simulink model "buck_conv"  (R2020b)
settings: Solver=ode3  StartTime=0.0  StopTime=0.06  FixedStep=1e-7  RelTol=1e-3  EnableMultiTasking=on
undefined symbols (not defined in the file): C, ki, kp, L, R, T, Vin, Vo
libraries: simulink x3
settings Model: Creator=Anandarup  LastModifiedBy=Anandarup
settings DataIOCC: LimitDataPoints=on  SaveFormat=Array  ReturnWorkspaceOutputs=off
settings OptimizationCC: LifeSpan=inf
settings DebuggingCC: SolverPrmCheckMsg=warning  SFUnexpectedBacktrackingDiag=warning  SFNoUnconditionalDefaultTransitionDiag=warning  SFExecutionAtInitializationDiag=none  ArithmeticOperatorsInVariantConditions=warning
settings HardwareCC: ProdBitPerPointer=32  ProdBitPerSizeT=32  ProdBitPerPtrDiffT=32  ProdLargestAtomicFloat=None  ProdIntDivRoundTo=Undefined  ProdEndianess=Unspecified  ProdWordSize=32  ProdHWDeviceType=32-bit Generic
settings ModelReferenceCC: PropagateSignalLabelsOutOfModel=off
settings SFSimCC: SimUseLocalCustomCode=off  CustomCodeUndefinedFunction=UseInterfaceOnly
settings RTWCC: RTWUseLocalCustomCode=off
settings CodeAppCC: StateflowObjectComments=on
settings GRTTargetCC: TargetLangStandard=C89/C90 (ANSI)
settings ConfigComp: CovMetricSettings=dw  CovSaveCumulativeToWorkspaceVar=on  CovSaveSingleToWorkspaceVar=on  CovExternalEMLEnable=off  CovSFcnEnable=off

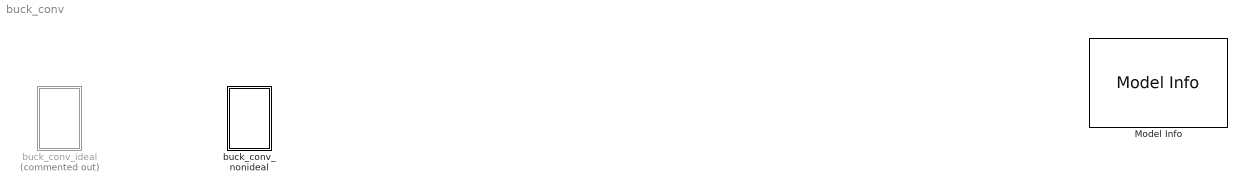
== system buck_conv ==
  Model Info : simulink/Model-Wide Utilities/Model Info  Frame=on  DisplayStringWithTags=|  HorizontalTextAlignment=Center  LeftAlignmentValue=0.5
      | clear;
      | clc;
      | R=5;
      | Vin=24;
      | L=750e-6;
      | C=1.5e-6;
      | Vo=15;
      | kp=20;
      | ki=10;
      | T=1/50e3;
  buck_conv_ideal : Subsystem  Commented=on
  buck_conv_nonideal : Subsystem

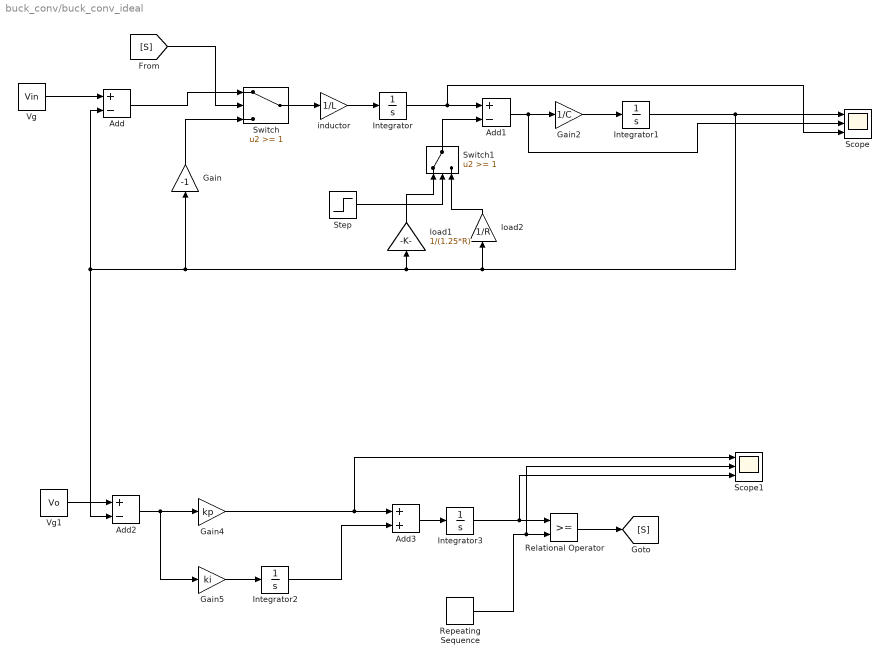
== system buck_conv/buck_conv_ideal ==
  Add : Sum  Inputs=+-
  Add1 : Sum  Inputs=+-
  Add2 : Sum  Inputs=+-
  Add3 : Sum  Inputs=2
  Gain : Gain  Gain=-1
  Gain2 : Gain  Gain=1/C
  Gain4 : Gain  Gain=kp
  Gain5 : Gain  Gain=ki
  Integrator : Integrator
  Integrator1 : Integrator
  Integrator2 : Integrator  LimitOutput=on  UpperSaturationLimit=1  LowerSaturationLimit=-1
  Integrator3 : Integrator  LimitOutput=on  UpperSaturationLimit=1  LowerSaturationLimit=-1
  Relational Operator : RelationalOperator  OutDataTypeStr=boolean  RndMeth=Nearest
  Repeating Sequence : simulink/Sources/Repeating Sequence  rep_seq_t=[0 0.5*T T]  rep_seq_y=[0 1 0]
  Scope : Scope  NumInputPorts=3
  Scope1 : Scope  NumInputPorts=3
  Step : Step  Time=0.03  SampleTime=0
  Switch : Switch  Threshold=1
  Switch1 : Switch  Threshold=1
  Vg : Constant  Value=Vin
  Vg1 : Constant  Value=Vo
  inductor : Gain  Gain=1/L
  load1 : Gain  Gain=1/(1.25*R)
  load2 : Gain  Gain=1/R
  wires:
  Gain2/1 -> Integrator1/1
  Add2/1 -> Gain5/1, Gain4/1
  Add1/1 -> Scope/2, Gain2/1
  Gain5/1 -> Integrator2/1
  Vg/1 -> Add/1
  Integrator1/1 -> Scope/1, load2/1, Add2/2, Add/2, Gain/1, load1/1
  Integrator/1 -> Scope/3, Add1/1
  Add/1 -> Switch/1
  Gain/1 -> Switch/3
  Integrator2/1 -> Add3/2
  Add3/1 -> Integrator3/1
  Gain4/1 -> Scope1/1, Add3/1
  Switch/1 -> inductor/1
  Integrator3/1 -> Scope1/3, Relational Operator/1
  Repeating Sequence/1 -> Scope1/2, Relational Operator/2
  Relational Operator/1 -> [S]
  Switch1/1 -> Add1/2
  load2/1 -> Switch1/3
  [S] -> Switch/2
  load1/1 -> Switch1/1
  Step/1 -> Switch1/2
  Vg1/1 -> Add2/1
  inductor/1 -> Integrator/1

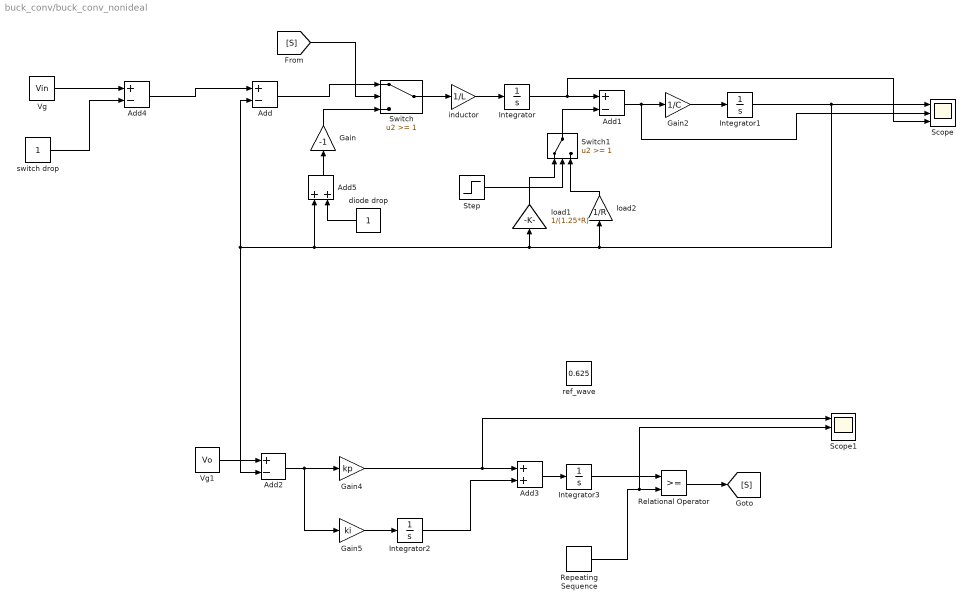
== system buck_conv/buck_conv_nonideal ==
  Add{,1..2,4} (4 alike) : Sum  Inputs=+-
  Add3 : Sum  Inputs=2
  Add5 : Sum  Inputs=2
  Gain : Gain  Gain=-1
  Gain2 : Gain  Gain=1/C
  Gain4 : Gain  Gain=kp
  Gain5 : Gain  Gain=ki
  Integrator : Integrator
  Integrator1 : Integrator
  Integrator2 : Integrator  LimitOutput=on  UpperSaturationLimit=1  LowerSaturationLimit=-1
  Integrator3 : Integrator  LimitOutput=on  UpperSaturationLimit=1  LowerSaturationLimit=-1
  Relational Operator : RelationalOperator  OutDataTypeStr=boolean  RndMeth=Nearest
  Repeating Sequence : simulink/Sources/Repeating Sequence  rep_seq_t=[0 0.5*T T]  rep_seq_y=[0 1 0]
  Scope : Scope  NumInputPorts=3
  Scope1 : Scope  NumInputPorts=3
  Step : Step  Time=0.03  SampleTime=0
  Switch : Switch  Threshold=1
  Switch1 : Switch  Threshold=1
  Vg : Constant  Value=Vin
  Vg1 : Constant  Value=Vo
  diode drop : Constant
  inductor : Gain  Gain=1/L
  load1 : Gain  Gain=1/(1.25*R)
  load2 : Gain  Gain=1/R
  ref_wave : Constant  Value=0.625
  switch drop : Constant
  wires:
  inductor/1 -> Integrator/1
  Vg1/1 -> Add2/1
  Step/1 -> Switch1/2
  load1/1 -> Switch1/1
  [S] -> Switch/2
  load2/1 -> Switch1/3
  Switch1/1 -> Add1/2
  Relational Operator/1 -> [S]
  Repeating Sequence/1 -> Relational Operator/2, Scope1/2
  Switch/1 -> inductor/1
  Gain4/1 -> Add3/1, Scope1/1
  Add3/1 -> Integrator3/1
  Integrator2/1 -> Add3/2
  Gain/1 -> Switch/3
  Add/1 -> Switch/1
  Integrator/1 -> Add1/1, Scope/3
  Integrator1/1 -> load1/1, Add5/1, Add/2, Add2/2, load2/1, Scope/1
  Gain5/1 -> Integrator2/1
  Add1/1 -> Gain2/1, Scope/2
  Add2/1 -> Gain4/1, Gain5/1
  Gain2/1 -> Integrator1/1
  Vg/1 -> Add4/1
  Add4/1 -> Add/1
  switch drop/1 -> Add4/2
  Add5/1 -> Gain/1
  diode drop/1 -> Add5/2
  Integrator3/1 -> Relational Operator/1
